simulink model "LCK_0112"  (R2018b)
settings: Solver=FixedStepDiscrete  StartTime=0.0  StopTime=inf  FixedStep=0.01  RelTol=1e-3
PostLoadFcn:
  | if any(exist('dsrtsu_mdlpostloadfcn', 'file') ~= 0), dsrtsu_mdlpostloadfcn('Execute', bdroot); end
values from neighbouring files (symbols this model uses):
  C_DEG2RAD = 0.0175    [LCK_Macro.sldd]
  C_KPH2MPS = 0.2778    [LCK_Macro.sldd]
  C_NEARZERO = 0.0001    [LCK_Macro.sldd]
  C_ONE = 1.0    [LCK_Macro.sldd]
  C_RAD2DEG = 57.2958    [LCK_Macro.sldd]
  C_ZERO = 0.0    [LCK_Macro.sldd]
  k_accel_pedal_pos_per_speed_x : value not decoded    [LCK_LogicPara.sldd]
  k_accel_pedal_pos_per_speed_z : value not decoded    [LCK_LogicPara.sldd]
  k_brake_suprress_hold = 1000.0    [LCK_LogicPara.sldd]
  k_driver_appl_torque_filt = 50.0    [LCK_LogicPara.sldd]
  k_driver_suppression_hold_time = 3000.0    [LCK_LogicPara.sldd]
  k_hands_on_wheel_hold_msec = 500.0    [LCK_LogicPara.sldd]
  k_hands_on_wheel_torque_hi = 0.2    [LCK_LogicPara.sldd]
  k_hands_on_wheel_torque_lo = 0.15    [LCK_LogicPara.sldd]
  k_handsoff_delay_cycles = 50.0    [LCK_LogicPara.sldd]
  k_handsoff_torq_Lo_CR = 0.3    [LCK_LogicPara.sldd]
  k_handson_delay_cycles = 5.0    [LCK_LogicPara.sldd]
  k_HighAccel_suppress_hold = 3000.0    [LCK_LogicPara.sldd]
  k_HLR_suprress_hold = 3000.0    [LCK_LogicPara.sldd]
  k_hs_StrAng_CR_threshold_z : value not decoded    [LCK_LogicPara.sldd]
  k_LC_Exit_Switch = 0.0    [LCK_LogicPara.sldd]
  k_LCG_Configured = 1.0    [LCK_LogicPara.sldd]
  k_LCK_A0_Rdy2Act_UseConst = 0.0    [LCK_LogicPara.sldd]
  k_LCK_A0Fac_ActSta : value not decoded    [LCK_CtrlPara.sldd]
  k_LCK_A0Fac_DrvStm : value not decoded    [LCK_CtrlPara.sldd]
  k_LCK_A0Shift_LftCurv : value not decoded    [LCK_CtrlPara.sldd]
  k_LCK_A0Shift_RgtCurv : value not decoded    [LCK_CtrlPara.sldd]
  k_LCK_A0Shift_StraLan = 0.0    [LCK_CtrlPara.sldd]
  k_LCK_A0ShiftFac_Dy_LftCurv : value not decoded    [LCK_CtrlPara.sldd]
  k_LCK_A0ShiftFac_Dy_RgtCurv : value not decoded    [LCK_CtrlPara.sldd]
  k_LCK_A0ShiftFac_Vspd : value not decoded    [LCK_CtrlPara.sldd]
  k_LCK_accel_inhibit_thold = 35.0    [LCK_LogicPara.sldd]
  k_LCK_Active2Ready_Mask = 255.0    [LCK_LogicPara.sldd]
  k_LCK_CvatRateBks : value not decoded    [LCK_CtrlPara.sldd]
  k_LCK_CvatrBks : value not decoded    [LCK_CtrlPara.sldd]
  k_LCK_DFac_Dy : value not decoded    [LCK_CtrlPara.sldd]
  k_LCK_DFac_Dy_Curv : value not decoded    [LCK_CtrlPara.sldd]
  k_LCK_DFac_HaCurCen : value not decoded    [LCK_CtrlPara.sldd]
  k_LCK_DFac_HaCurSid : value not decoded    [LCK_CtrlPara.sldd]
  k_LCK_DFac_HadCurCen : value not decoded    [LCK_CtrlPara.sldd]
  k_LCK_DFac_HadCurSid : value not decoded    [LCK_CtrlPara.sldd]
  k_LCK_DFac_HadStrCen : value not decoded    [LCK_CtrlPara.sldd]
  k_LCK_DFac_HadStrSid : value not decoded    [LCK_CtrlPara.sldd]
  k_LCK_DFac_HaStrCen : value not decoded    [LCK_CtrlPara.sldd]
  k_LCK_DFac_HaStrSid : value not decoded    [LCK_CtrlPara.sldd]
  k_LCK_DFac_Rad : value not decoded    [LCK_CtrlPara.sldd]
  k_LCK_DFac_SA_CurCen : value not decoded    [LCK_CtrlPara.sldd]
  k_LCK_DFac_SA_CurSid : value not decoded    [LCK_CtrlPara.sldd]
  k_LCK_DFac_SA_StrCen : value not decoded    [LCK_CtrlPara.sldd]
  k_LCK_DFac_SA_StrSid : value not decoded    [LCK_CtrlPara.sldd]
  k_LCK_DFac_SS_CurCen : value not decoded    [LCK_CtrlPara.sldd]
  k_LCK_DFac_SS_CurSid : value not decoded    [LCK_CtrlPara.sldd]
  k_LCK_DFac_SS_StrCen : value not decoded    [LCK_CtrlPara.sldd]
  k_LCK_DFac_SS_StrSid : value not decoded    [LCK_CtrlPara.sldd]
  k_LCK_DFac_Vspd : value not decoded    [LCK_CtrlPara.sldd]
  k_LCK_DlyTm_DrvStim = 0.2    [LCK_CtrlPara.sldd]
  k_LCK_DTermMax = 2.0    [LCK_CtrlPara.sldd]
  k_LCK_DyBks_Curv : value not decoded    [LCK_CtrlPara.sldd]
  k_LCK_Enable_POOnly = 1.0    [LCK_LogicPara.sldd]
  k_LCK_Entry_DistBuffer = 0.1    [LCK_LogicPara.sldd]
  k_LCK_Fac_Vspd2RngThr_FalRec = 0.23    [LCK_CtrlPara.sldd]
  k_LCK_Ffw_CvatSwh = 0.0    [LCK_CtrlPara.sldd]
  k_LCK_Ffw_DyBks : value not decoded    [LCK_CtrlPara.sldd]
  k_LCK_Ffw_TimCon_CmdFlt = 0.0    [LCK_CtrlPara.sldd]
  k_LCK_FfwDeltaFac_Rad_Lft : value not decoded    [LCK_CtrlPara.sldd]
  k_LCK_FfwDeltaFac_Rad_Rgt : value not decoded    [LCK_CtrlPara.sldd]
  k_LCK_FfwDeltaFac_Vspd : value not decoded    [LCK_CtrlPara.sldd]
  k_LCK_FfwFac_CvatRate_Lft : value not decoded    [LCK_CtrlPara.sldd]
  k_LCK_FfwFac_CvatRate_Rgt : value not decoded    [LCK_CtrlPara.sldd]
  k_LCK_FfwFac_Dy : value not decoded    [LCK_CtrlPara.sldd]
  k_LCK_FfwFac_Rad_Lft : value not decoded    [LCK_CtrlPara.sldd]
  k_LCK_FfwFac_Rad_Rgt : value not decoded    [LCK_CtrlPara.sldd]
  k_LCK_FfwFac_Vspd : value not decoded    [LCK_CtrlPara.sldd]
  k_LCK_FfwTorq_Cvat : value not decoded    [LCK_CtrlPara.sldd]
  k_LCK_HAFac_ActSta : value not decoded    [LCK_CtrlPara.sldd]
  k_LCK_HAFac_DrvStm : value not decoded    [LCK_CtrlPara.sldd]
  k_LCK_HaloTime = 2000.0    [LCK_LogicPara.sldd]
  k_LCK_HaloTime_Switch = 0.0    [LCK_LogicPara.sldd]
  k_LCK_HARFac_ActSta : value not decoded    [LCK_CtrlPara.sldd]
  k_LCK_HARFac_DrvStm : value not decoded    [LCK_CtrlPara.sldd]
  k_LCK_Hed_DyBks : value not decoded    [LCK_CtrlPara.sldd]
  k_LCK_HedAngDiffX : value not decoded    [LCK_CtrlPara.sldd]
  k_LCK_HedAngRateDiffX : value not decoded    [LCK_CtrlPara.sldd]
  k_LCK_HndsOnWhel_DlyTm_Idl2Rdy = 0.0    [LCK_LogicPara.sldd]
  k_LCK_host_veh_width = 1.86    [LCK_LogicPara.sldd]
  k_LCK_Idle2Ready_Mask = 239.0    [LCK_LogicPara.sldd]
  k_LCK_Junc_SusTime = 1.0    [LCK_LogicPara.sldd]
  k_LCK_KpKdDecSlopeLmt = 10.0    [LCK_CtrlPara.sldd]
  k_LCK_KpKdIncSlopeLmt = 5.0    [LCK_CtrlPara.sldd]
  k_LCK_Lat_Ctrl_DFac_Lft = 1.0    [LCK_CtrlPara.sldd]
  k_LCK_Lat_Ctrl_DFac_Rgt = 1.05    [LCK_CtrlPara.sldd]
  k_LCK_Lat_Ctrl_Kd = 0.8    [LCK_CtrlPara.sldd]
  k_LCK_Lat_Ctrl_Ki = 0.5    [LCK_CtrlPara.sldd]
  k_LCK_Lat_Ctrl_Kp = 0.7    [LCK_CtrlPara.sldd]
  k_LCK_Lat_Ctrl_Kp_NearGain = 0.7    [LCK_CtrlPara.sldd]
  k_LCK_Lat_Ctrl_PFac_Lft = 1.0    [LCK_CtrlPara.sldd]
  k_LCK_Lat_Ctrl_PFac_Rgt = 1.05    [LCK_CtrlPara.sldd]
  k_LCK_Lat_Ctrl_TimCon_CmdFlt = 5.0    [LCK_CtrlPara.sldd]
  k_LCK_Lat_DFac_Rad : value not decoded    [LCK_CtrlPara.sldd]
  k_LCK_Lat_DFac_SS_Cur : value not decoded    [LCK_CtrlPara.sldd]
  k_LCK_Lat_DFac_SS_Str : value not decoded    [LCK_CtrlPara.sldd]
  k_LCK_Lat_DFac_Vspd : value not decoded    [LCK_CtrlPara.sldd]
  k_LCK_Lat_DyBks : value not decoded    [LCK_CtrlPara.sldd]
  k_LCK_Lat_IFac_Rad : value not decoded    [LCK_CtrlPara.sldd]
  k_LCK_Lat_IFac_Vspd : value not decoded    [LCK_CtrlPara.sldd]
  k_LCK_Lat_ILmtFac_Dy_CurvLan : value not decoded    [LCK_CtrlPara.sldd]
  k_LCK_Lat_ILmtFac_Dy_StraLan : value not decoded    [LCK_CtrlPara.sldd]
  k_LCK_Lat_ILmtFac_Rad : value not decoded    [LCK_CtrlPara.sldd]
  k_LCK_Lat_ILmtFac_Rad_NearGain = 1.0    [LCK_CtrlPara.sldd]
  k_LCK_Lat_ILmtFac_Vspd_CurvLan : value not decoded    [LCK_CtrlPara.sldd]
  k_LCK_Lat_ILmtFac_Vspd_StraLan : value not decoded    [LCK_CtrlPara.sldd]
  k_LCK_Lat_ITermLmt_Dy = 1.0    [LCK_CtrlPara.sldd]
  k_LCK_Lat_KpKdDecSlopeLmt = 10.0    [LCK_CtrlPara.sldd]
  k_LCK_Lat_KpKdIncSlopeLmt = 10.0    [LCK_CtrlPara.sldd]
  k_LCK_Lat_PFac_Dy_InnLftCur : value not decoded    [LCK_CtrlPara.sldd]
  k_LCK_Lat_PFac_Dy_InnRgtCur : value not decoded    [LCK_CtrlPara.sldd]
  k_LCK_Lat_PFac_Dy_OutLftCur : value not decoded    [LCK_CtrlPara.sldd]
  k_LCK_Lat_PFac_Dy_OutRgtCur : value not decoded    [LCK_CtrlPara.sldd]
  k_LCK_Lat_PFac_Dy_Str : value not decoded    [LCK_CtrlPara.sldd]
  k_LCK_Lat_PFac_Rad : value not decoded    [LCK_CtrlPara.sldd]
  ... (+153 more)
undefined symbols (not defined in the file or in its folder): k_LCK_CurvBks, K_LCK_SPA0A1A2_LMRngCmp_y
libraries: LateralControl_fcns_lib x58, simulink x24
(part 34 of 45)

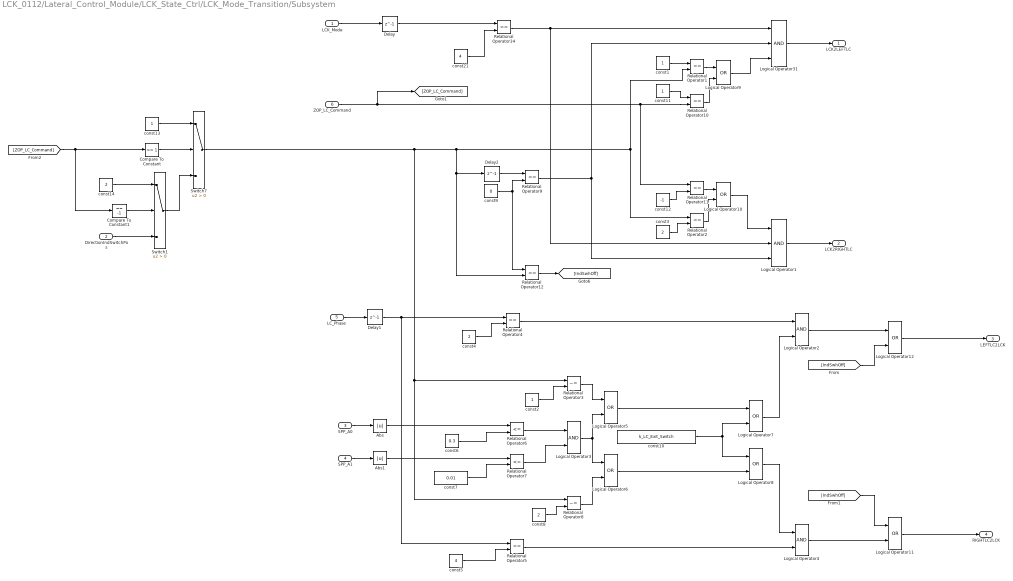
== system LCK_0112/Lateral_Control_Module/LCK_State_Ctrl/LCK_Mode_Transition/Subsystem ==
  LCK_Mode : Inport
  DirectionIndSwitchPos : Inport  Port=2
  SPP_A0 : Inport  Port=3
  SPP_A1 : Inport  Port=4
  LC_Phase : Inport  Port=5
  ZOP_LC_Command : Inport  Port=6
  Abs : Abs
  Abs1 : Abs
  Compare To Constant : simulink/Logic and Bit Operations/Compare To Constant  relop===  const=1  OutDataTypeStr=boolean
  Compare To Constant1 : simulink/Logic and Bit Operations/Compare To Constant  relop===  const=-1  OutDataTypeStr=boolean
  Delay : Delay  DelayLength=1  InitialCondition=0
  Delay1 : Delay  DelayLength=1  InitialCondition=0
  Delay2 : Delay  DelayLength=1  InitialCondition=0
  Logical Operator1 : Logic  Tag={'date',737237.63746706024}  Description=_GWMAB30P3.LCK.000_65_  Inputs=3  AllPortsSameDT=off  OutDataTypeStr=boolean
  Logical Operator{5..12} (8 alike) : Logic  Tag={'date',737237.63746706024}  Description=_GWMAB30P3.LCK.000_65_  Operator=OR  AllPortsSameDT=off  OutDataTypeStr=boolean
  Logical Operator2 : Logic  Tag={'date',737237.63746706024}  Description=_GWMAB30P3.LCK.000_65_  AllPortsSameDT=off  OutDataTypeStr=boolean
  Logical Operator3 : Logic  Tag={'date',737237.63746706024}  Description=_GWMAB30P3.LCK.000_65_  AllPortsSameDT=off  OutDataTypeStr=boolean
  Logical Operator31 : Logic  Tag={'date',737237.63746706024}  Description=_GWMAB30P3.LCK.000_65_  Inputs=3  AllPortsSameDT=off  OutDataTypeStr=boolean
  Logical Operator4 : Logic  Tag={'date',737237.63746706024}  Description=_GWMAB30P3.LCK.000_65_  AllPortsSameDT=off  OutDataTypeStr=boolean
  Relational Operator{1..2,4..5,9..12,34} (9 alike) : RelationalOperator  Tag={'date',737237.63747177087}  Description=_GWMAB30P3.LCK.000_91_  Operator===  OutDataTypeStr=boolean  RndMeth=Nearest
  Relational Operator3 : RelationalOperator  Tag={'date',737237.63747177087}  Description=_GWMAB30P3.LCK.000_91_  Operator=~=  OutDataTypeStr=boolean  RndMeth=Nearest
  Relational Operator6 : RelationalOperator  Tag={'date',737237.63747177087}  Description=_GWMAB30P3.LCK.000_91_  Operator=<=  OutDataTypeStr=boolean  RndMeth=Nearest
  Relational Operator7 : RelationalOperator  Tag={'date',737237.63747177087}  Description=_GWMAB30P3.LCK.000_91_  Operator=<=  OutDataTypeStr=boolean  RndMeth=Nearest
  Relational Operator8 : RelationalOperator  Tag={'date',737237.63747177087}  Description=_GWMAB30P3.LCK.000_91_  Operator=~=  OutDataTypeStr=boolean  RndMeth=Nearest
  Switch1 : Switch  Criteria=u2 > Threshold
  Switch7 : Switch  Criteria=u2 > Threshold
  const{1..2,11,13} (4 alike) : Constant  Tag={'output',{'type','Int32'},'date',737237.63747863425}  Description=_GWMAB30P3.LCK.000_128_
  const10 : Constant  Tag={'output',{'type','Int32'},'date',737237.63747863425}  Description=_GWMAB30P3.LCK.000_128_  Value=k_LC_Exit_Switch
  const12 : Constant  Tag={'output',{'type','Int32'},'date',737237.63747863425}  Description=_GWMAB30P3.LCK.000_128_  Value=-1
  const{3..4,8,14} (4 alike) : Constant  Tag={'output',{'type','Int32'},'date',737237.63747863425}  Description=_GWMAB30P3.LCK.000_128_  Value=2
  const21 : Constant  Tag={'output',{'type','Int32'},'date',737237.63747863425}  Description=_GWMAB30P3.LCK.000_128_  Value=4
  const5 : Constant  Tag={'output',{'type','Int32'},'date',737237.63747863425}  Description=_GWMAB30P3.LCK.000_128_  Value=4
  const6 : Constant  Tag={'output',{'type','Int32'},'date',737237.63747863425}  Description=_GWMAB30P3.LCK.000_128_  Value=0.3
  const7 : Constant  Tag={'output',{'type','Int32'},'date',737237.63747863425}  Description=_GWMAB30P3.LCK.000_128_  Value=0.01
  const9 : Constant  Tag={'output',{'type','Int32'},'date',737237.63747863425}  Description=_GWMAB30P3.LCK.000_128_  Value=0
  LCK2LEFTLC : Outport
  LCK2RIGHTLC : Outport  Port=2
  LEFTLC2LCK : Outport  Port=3
  RIGHTLC2LCK : Outport  Port=4
  wires:
  Relational Operator34/1 -> Logical Operator31/1, Logical Operator1/2
  const1/1 -> Relational Operator1/1
  LCK_Mode/1 -> Delay/1
  const21/1 -> Relational Operator34/2
  const3/1 -> Relational Operator2/2
  Delay/1 -> Relational Operator34/1
  Logical Operator31/1 -> LCK2LEFTLC/1
  Logical Operator1/1 -> LCK2RIGHTLC/1
  Relational Operator4/1 -> Logical Operator2/1
  const4/1 -> Relational Operator4/2
  const5/1 -> Relational Operator5/2
  SPP_A0/1 -> Abs/1
  const6/1 -> Relational Operator6/2
  SPP_A1/1 -> Abs1/1
  const7/1 -> Relational Operator7/2
  Relational Operator6/1 -> Logical Operator3/1
  Relational Operator7/1 -> Logical Operator3/2
  LC_Phase/1 -> Delay1/1
  Relational Operator5/1 -> Logical Operator4/2
  Delay1/1 -> Relational Operator4/1, Relational Operator5/1
  Abs1/1 -> Relational Operator7/1
  Abs/1 -> Relational Operator6/1
  const2/1 -> Relational Operator3/2
  Relational Operator3/1 -> Logical Operator5/1
  Logical Operator3/1 -> Logical Operator6/1, Logical Operator5/2
  const8/1 -> Relational Operator8/2
  Relational Operator8/1 -> Logical Operator6/2
  Delay2/1 -> Relational Operator9/1
  Relational Operator9/1 -> Logical Operator31/2, Logical Operator1/3
  Logical Operator5/1 -> Logical Operator7/1
  const10/1 -> Logical Operator8/1, Logical Operator7/2
  Logical Operator7/1 -> Logical Operator2/2
  Logical Operator6/1 -> Logical Operator8/2
  Logical Operator8/1 -> Logical Operator4/1
  Relational Operator1/1 -> Logical Operator9/1
  ZOP_LC_Command/1 -> [ZOP_LC_Command], Relational Operator10/2, Relational Operator11/1
  Relational Operator10/1 -> Logical Operator9/2
  Relational Operator11/1 -> Logical Operator10/1
  Relational Operator2/1 -> Logical Operator10/2
  Logical Operator10/1 -> Logical Operator1/1
  Logical Operator9/1 -> Logical Operator31/3
  const12/1 -> Relational Operator11/2
  const11/1 -> Relational Operator10/1
  [IndSwhOff] -> Logical Operator12/2
  Relational Operator12/1 -> [IndSwhOff]
  [IndSwhOff] -> Logical Operator11/1
  Switch7/1 -> Relational Operator8/1, Relational Operator3/1, Relational Operator12/2, Delay2/1, Relational Operator2/1, Relational Operator1/2
  const9/1 -> Relational Operator12/1, Relational Operator9/2
  Logical Operator2/1 -> Logical Operator12/1
  Logical Operator12/1 -> LEFTLC2LCK/1
  Logical Operator4/1 -> Logical Operator11/2
  Logical Operator11/1 -> RIGHTLC2LCK/1
  [ZOP_LC_Command] -> Compare To Constant1/1, Compare To Constant/1
  Compare To Constant/1 -> Switch7/2
  const13/1 -> Switch7/1
  Compare To Constant1/1 -> Switch1/2
  const14/1 -> Switch1/1
  Switch1/1 -> Switch7/3
  DirectionIndSwitchPos/1 -> Switch1/3
